simulink model "ARDroneWPTracking"  (R2014a)
settings: Solver=ode1  StartTime=0.0  StopTime=inf  FixedStep=sampleTime  RelTol=1e-3
values from neighbouring files (symbols this model uses):
  sampleTime = 0.04    [start.m]
  waypoints = getWaypoints()    [start.m]
undefined symbols (not defined in the file or in its folder): Standard_Devices, UDP_Protocol
libraries: ARBlocks x2, rtwinlib x1
CloseFcn:
  | rtwprivate ssgencode ModelCloseRequest Good_NL_model
settings Model: SimulationMode=external  ExtModeTrigDuration=100000  Creator=Paul  LastModifiedBy=Django
settings DataIOCC: SignalLoggingSaveFormat=ModelDataLogs  TimeSaveName=time
settings OptimizationCC: ExpressionDepthLimit=2147483647  InitFltsAndDblsToZero=on
settings DebuggingCC: UnderspecifiedInitializationDetection=Classic  FcnCallInpInsideContextMsg=UseLocalSettings  StateNameClashWarn=warning
settings HardwareCC: ProdIntDivRoundTo=Zero  ProdEndianess=LittleEndian  ProdHWDeviceType=Generic->32-bit x86 compatible
settings RTWCC: SystemTargetFile=rtwin.tlc  TemplateMakefile=rtwin.tmf  Description=Real-Time Windows Target  ProcessScript=rtwin_make_rtw_hook  RTWCompilerOptimization=On
settings CodeAppCC: MaxIdLength=95
settings RTWinTargetCC: TargetLibSuffix=_rtwin.lib  TargetPreCompLibLocation=E:\Installationposition\InstallPath\MATLAB\MATLAB2014a\toolbox\rtw\targets\rtwin\lib\win64

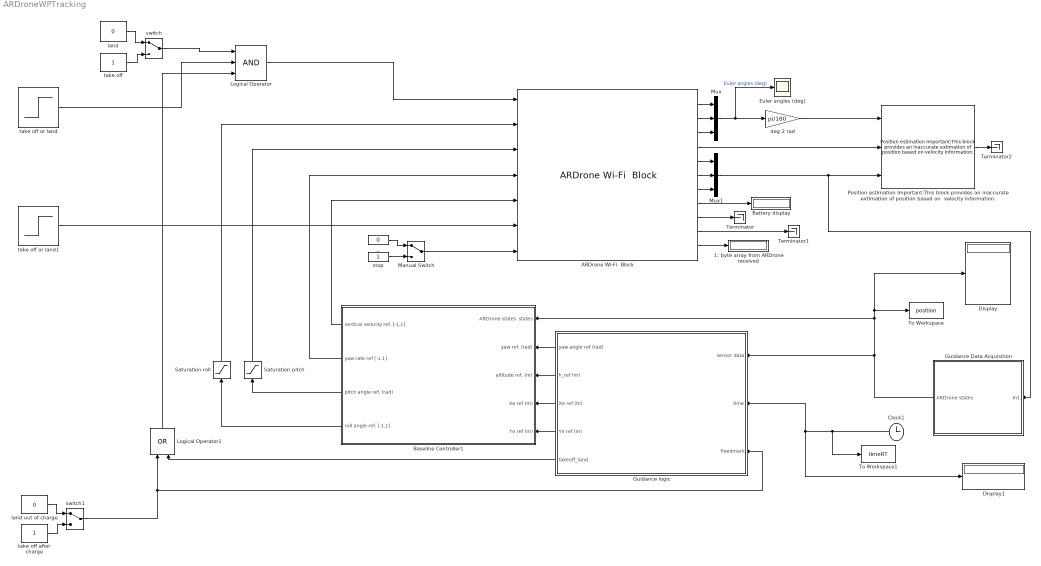
== system ARDroneWPTracking ==
  "1: byte array from ARDrone received " : Display
  ARDrone Wi-Fi  Block : ARBlocks/ARDrone Wi-Fi  Block
  Baseline Controller1 : Subsystem  AncestorBlock=ARBlocks/Baseline Controller
  Battery display : Display
  Clock1 : Clock
  Display : Display
  Display1 : Display
  Euler angles (deg) : Scope
      settings: YMin=-10  YMax=120  MaxDataPoints=500000
  Guidance Data Acquisition : Subsystem  AncestorBlock=ARBlocks/Guidance Data Acquisition
  Guidance logic : Subsystem  AncestorBlock=ARBlocks/Guidance logic
  Logical Operator : Logic  Inputs=3  AllPortsSameDT=off  OutDataTypeStr=boolean
  Logical Operator1 : Logic  Operator=OR  AllPortsSameDT=off  OutDataTypeStr=boolean
  Manual Switch : ManualSwitch
  Mux : Mux  Inputs=3
  Mux1 : Mux  Inputs=3
  "Position estimation Important:This block provides an inaccurate extimation of position based on  velocity information. " : ARBlocks/Position estimation Important:This block provides an  inaccurate extimation of position  based on  velocity information. 
  Saturation pitch : Saturate  UpperLimit=0.08  LowerLimit=-0.1
  Saturation roll : Saturate  UpperLimit=0.05  LowerLimit=-0.1
  Terminator : Terminator
  Terminator1 : Terminator
  Terminator2 : Terminator
  To Workspace : ToWorkspace  VariableName=position  SaveFormat=Structure With Time  SampleTime=sampleTime
  To Workspace1 : ToWorkspace  VariableName=timeRT  SampleTime=sampleTime
  _ : Constant  Value=0
  deg 2 rad : Gain  Gain=pi/180
  land : Constant  Value=0
  land out of charge : Constant  Value=0
  stop : Constant
  switch : ManualSwitch
  switch1 : ManualSwitch
  take off : Constant
  take off after charge : Constant
  take off or land : Step  Time=5  SampleTime=0
  take off or land1 : Step  Time=10  SampleTime=0
  wires:
  _/1 -> Manual Switch/1
  stop/1 -> Manual Switch/2
  Logical Operator/1 -> ARDrone Wi-Fi  Block/1
  take off or land1/1 -> ARDrone Wi-Fi  Block/6
  Manual Switch/1 -> ARDrone Wi-Fi  Block/7
  ARDrone Wi-Fi  Block/1 -> Mux/1
  ARDrone Wi-Fi  Block/2 -> Mux/2
  ARDrone Wi-Fi  Block/5 -> Mux1/1
  ARDrone Wi-Fi  Block/6 -> Mux1/2
  ARDrone Wi-Fi  Block/7 -> Mux1/3
  Mux/1 -> Euler angles (deg)/1, deg 2 rad/1  "Euler angles (deg)"
  ARDrone Wi-Fi  Block/8 -> Battery display/1
  Baseline Controller1/1(vertical velocity ref. [-1,1]) -> ARDrone Wi-Fi  Block/5
  Baseline Controller1/3(pitch angle ref. (rad)) -> Saturation pitch/1
  "Position estimation Important:This block provides an inaccurate extimation of position based on  velocity information. "/1 -> Terminator2/1
  deg 2 rad/1 -> "Position estimation Important:This block provides an inaccurate extimation of position based on  velocity information. "/1
  ARDrone Wi-Fi  Block/4 -> "Position estimation Important:This block provides an inaccurate extimation of position based on  velocity information. "/2
  Mux1/1 -> Guidance Data Acquisition/1(In1), "Position estimation Important:This block provides an inaccurate extimation of position based on  velocity information. "/3
  Clock1/1 -> To Workspace1/1, Display1/1, Guidance logic/2(time)
  Baseline Controller1/4(roll angle ref. [-1,1]) -> Saturation roll/1
  ARDrone Wi-Fi  Block/3 -> Mux/3
  Guidance logic/2(h_ref (m)) -> Baseline Controller1/3(altitude ref. (m))
  Guidance logic/4(Ye ref (m)) -> Baseline Controller1/5(Ye ref (m))
  Guidance logic/1(yaw angle ref (rad)) -> Baseline Controller1/2(yaw ref. (rad))
  ARDrone Wi-Fi  Block/9 -> Terminator/1
  ARDrone Wi-Fi  Block/10 -> Terminator1/1
  ARDrone Wi-Fi  Block/11 -> "1: byte array from ARDrone received "/1
  Baseline Controller1/2(yaw rate ref [-1,1]) -> ARDrone Wi-Fi  Block/4
  Guidance Data Acquisition/1(ARDrone states) -> Guidance logic/1(sensor data), Baseline Controller1/1("ARDrone states  states "), Display/1, To Workspace/1
  land/1 -> switch/1
  take off/1 -> switch/2
  switch/1 -> Logical Operator/1
  take off or land/1 -> Logical Operator/2
  Guidance logic/3(Xe ref (m)) -> Baseline Controller1/4(Xe ref (m))
  Logical Operator1/1 -> Logical Operator/3
  Saturation pitch/1 -> ARDrone Wi-Fi  Block/3
  Saturation roll/1 -> ARDrone Wi-Fi  Block/2
  land out of charge/1 -> switch1/1
  take off after charge/1 -> switch1/2
  switch1/1 -> Logical Operator1/1, Guidance logic/3(fixedmark)
  Guidance logic/5(takeoff_land) -> Logical Operator1/2

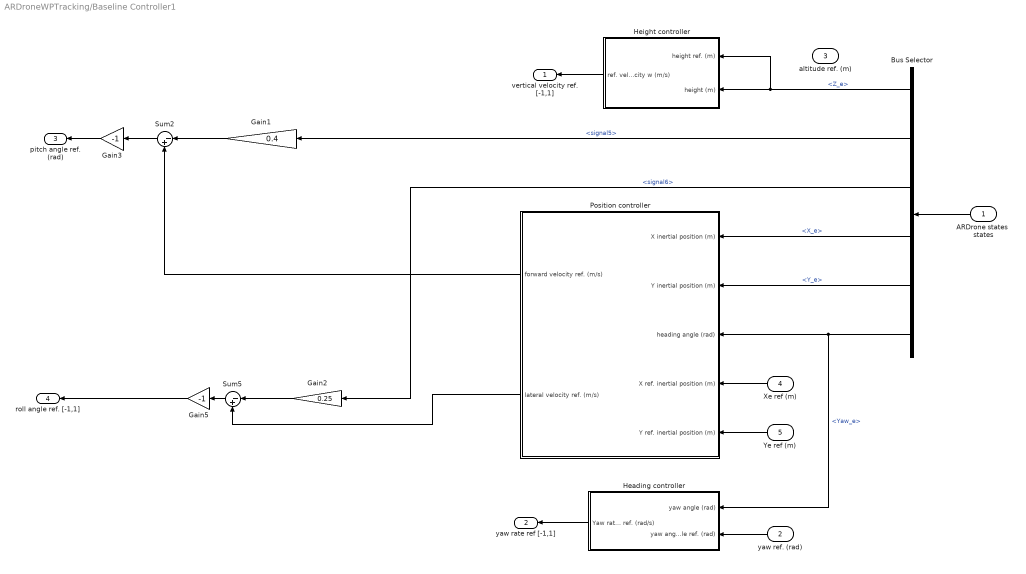
== system ARDroneWPTracking/Baseline Controller1 ==
  "ARDrone states  states " : Inport
  yaw ref. (rad) : Inport  Port=2
  altitude ref. (m) : Inport  Port=3
  Xe ref (m) : Inport  Port=4
  Ye ref (m) : Inport  Port=5
  Bus Selector : BusSelector  OutputSignals=Z_e,signal5,signal6,X_e,Y_e,Yaw_e
  Gain1 : Gain  Gain=0.4
  Gain2 : Gain  Gain=0.25
  Gain3 : Gain  Gain=-1
  Gain5 : Gain  Gain=-1
  Heading controller : Subsystem
  "Height controller " : Subsystem
  Position controller : Subsystem
  Sum2 : Sum  Inputs=|-+
  Sum5 : Sum  Inputs=|-+
  vertical velocity ref. [-1,1] : Outport
  yaw rate ref [-1,1] : Outport  Port=2
  pitch angle ref. (rad) : Outport  Port=3
  roll angle ref. [-1,1] : Outport  Port=4
  wires:
  Ye ref (m)/1 -> Position controller/5(Y ref. inertial position (m))
  Xe ref (m)/1 -> Position controller/4(X ref. inertial position (m))
  Bus Selector/5 -> Position controller/2(Y inertial position (m))  "<Y_e>"
  Bus Selector/4 -> Position controller/1(X inertial position (m))  "<X_e>"
  Heading controller/1(Yaw rate ref. (rad/s)) -> yaw rate ref [-1,1]/1
  yaw ref. (rad)/1 -> Heading controller/2(yaw angle ref. (rad))
  Bus Selector/2 -> Gain1/1  "<signal5>"
  Gain5/1 -> roll angle ref. [-1,1]/1
  "Height controller "/1(ref. velocity w (m/s)) -> vertical velocity ref. [-1,1]/1
  Bus Selector/1 -> "Height controller "/1(height ref. (m)), "Height controller "/2(height (m))  "<Z_e>"
  "ARDrone states  states "/1 -> Bus Selector/1
  Bus Selector/6 -> Position controller/3(heading angle (rad)), Heading controller/1(yaw angle (rad))  "<Yaw_e>"
  Sum2/1 -> Gain3/1
  Gain1/1 -> Sum2/1
  Gain3/1 -> pitch angle ref. (rad)/1
  Position controller/1(forward velocity ref. (m/s)) -> Sum2/2
  Sum5/1 -> Gain5/1
  Bus Selector/3 -> Gain2/1  "<signal6>"
  Gain2/1 -> Sum5/1
  Position controller/2(lateral velocity ref. (m/s)) -> Sum5/2

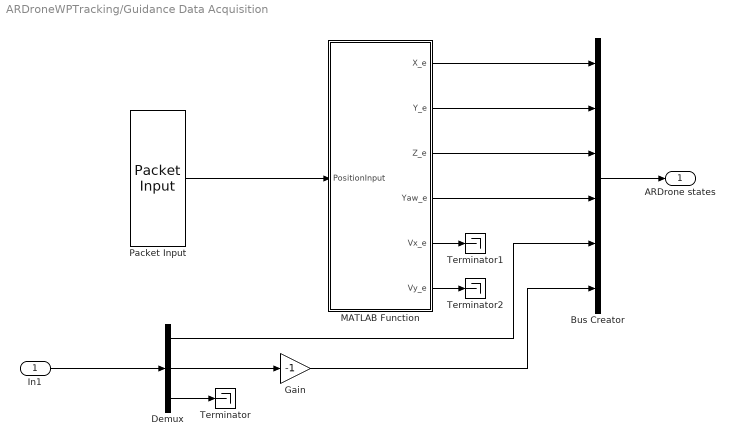
== system ARDroneWPTracking/Guidance Data Acquisition ==
  In1 : Inport
  Bus Creator : BusCreator  Inputs=6
  Demux : Demux  Outputs=3
  Gain : Gain  Gain=-1
  MATLAB Function : MATLAB Function  TreatAsAtomicUnit=on
  Packet Input : rtwinlib/Packet Input  SampleTime=sampleTime  MaxMissedTicks=1  ShowMissedTicks=off  YieldWhenWaiting=on  DrvName=Standard_Devices/UDP_Protocol  DrvAddress=5500  DrvOptions=[3215458314 5500]  PacketSize=32  DataTypes='4*double'  ShowReady=off  ShowError=off  PacketID=1  ByteOrder=2  ShowTimestamp=off
      settings: AttributesFormatString=Standard Devices\nUDP Protocol [157Ch]
  Terminator : Terminator
  Terminator1 : Terminator
  Terminator2 : Terminator
  ARDrone states : Outport
  wires:
  Demux/3 -> Terminator/1
  Demux/2 -> Gain/1
  In1/1 -> Demux/1
  Gain/1 -> Bus Creator/6
  Demux/1 -> Bus Creator/5
  Bus Creator/1 -> ARDrone states/1
  MATLAB Function/4(Yaw_e) -> Bus Creator/4
  Packet Input/1 -> MATLAB Function/1(PositionInput)
  MATLAB Function/1(X_e) -> Bus Creator/1
  MATLAB Function/2(Y_e) -> Bus Creator/2
  MATLAB Function/3(Z_e) -> Bus Creator/3
  MATLAB Function/5(Vx_e) -> Terminator1/1
  MATLAB Function/6(Vy_e) -> Terminator2/1

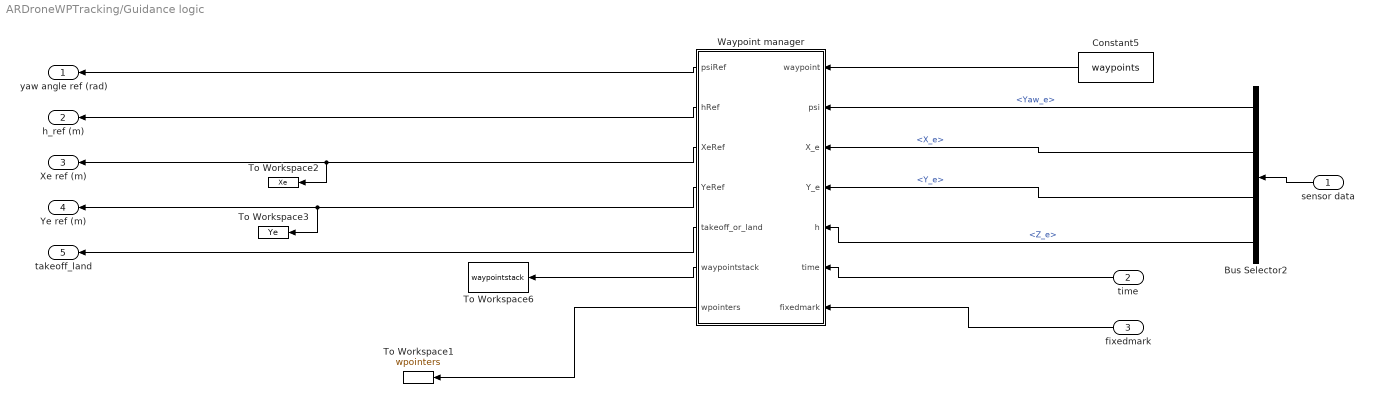
== system ARDroneWPTracking/Guidance logic ==
  sensor data : Inport
  time : Inport  Port=2
  fixedmark : Inport  Port=3
  Bus Selector2 : BusSelector  OutputSignals=Yaw_e,X_e,Y_e,Z_e
  Constant5 : Constant  Value=waypoints  VectorParams1D=off
  To Workspace1 : ToWorkspace  VariableName=wpointers  SampleTime=sampleTime
  To Workspace2 : ToWorkspace  VariableName=Xe  SampleTime=sampleTime
  To Workspace3 : ToWorkspace  VariableName=Ye  SampleTime=sampleTime
  To Workspace6 : ToWorkspace  VariableName=waypointstack  SampleTime=sampleTime
  "Waypoint manager " : MATLAB Function  TreatAsAtomicUnit=on
  yaw angle ref (rad) : Outport
  h_ref (m) : Outport  Port=2
  Xe ref (m) : Outport  Port=3
  Ye ref (m) : Outport  Port=4
  takeoff_land : Outport  Port=5
  wires:
  Constant5/1 -> "Waypoint manager "/1(waypoint)
  "Waypoint manager "/1(psiRef) -> yaw angle ref (rad)/1
  time/1 -> "Waypoint manager "/6(time)
  Bus Selector2/4 -> "Waypoint manager "/5(h)  "<Z_e>"
  "Waypoint manager "/4(YeRef) -> To Workspace3/1, Ye ref (m)/1
  "Waypoint manager "/3(XeRef) -> To Workspace2/1, Xe ref (m)/1
  "Waypoint manager "/2(hRef) -> h_ref (m)/1
  Bus Selector2/1 -> "Waypoint manager "/2(psi)  "<Yaw_e>"
  sensor data/1 -> Bus Selector2/1
  Bus Selector2/3 -> "Waypoint manager "/4(Y_e)  "<Y_e>"
  Bus Selector2/2 -> "Waypoint manager "/3(X_e)  "<X_e>"
  "Waypoint manager "/5(takeoff_or_land) -> takeoff_land/1
  "Waypoint manager "/6(waypointstack) -> To Workspace6/1
  fixedmark/1 -> "Waypoint manager "/7(fixedmark)
  "Waypoint manager "/7(wpointers) -> To Workspace1/1

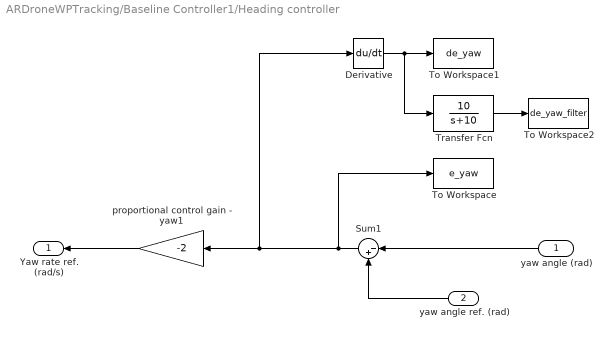
== system ARDroneWPTracking/Baseline Controller1/Heading controller ==
  yaw angle (rad) : Inport
  yaw angle ref. (rad) : Inport  Port=2
  Derivative : Derivative
  Sum1 : Sum  Inputs=|-+
  To Workspace : ToWorkspace  VariableName=e_yaw  SampleTime=-1
  To Workspace1 : ToWorkspace  VariableName=de_yaw  SampleTime=-1
  To Workspace2 : ToWorkspace  VariableName=de_yaw_filter  SampleTime=-1
  Transfer Fcn : TransferFcn  Numerator=[10]  Denominator=[1 10]
  proportional control gain - yaw1 : Gain  Gain=-2
  Yaw rate ref. (rad/s) : Outport
  wires:
  yaw angle ref. (rad)/1 -> Sum1/2
  yaw angle (rad)/1 -> Sum1/1
  proportional control gain - yaw1/1 -> Yaw rate ref. (rad/s)/1
  Sum1/1 -> proportional control gain - yaw1/1, Derivative/1, To Workspace/1
  Derivative/1 -> Transfer Fcn/1, To Workspace1/1
  Transfer Fcn/1 -> To Workspace2/1

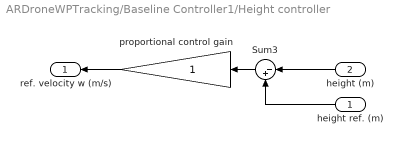
== system ARDroneWPTracking/Baseline Controller1/Height controller  ==
  height ref. (m) : Inport
  height (m) : Inport  Port=2
  Sum3 : Sum  Inputs=|-+
  proportional control gain : Gain
  ref. velocity w (m/s) : Outport
  wires:
  height ref. (m)/1 -> Sum3/2
  height (m)/1 -> Sum3/1
  Sum3/1 -> proportional control gain/1
  proportional control gain/1 -> ref. velocity w (m/s)/1

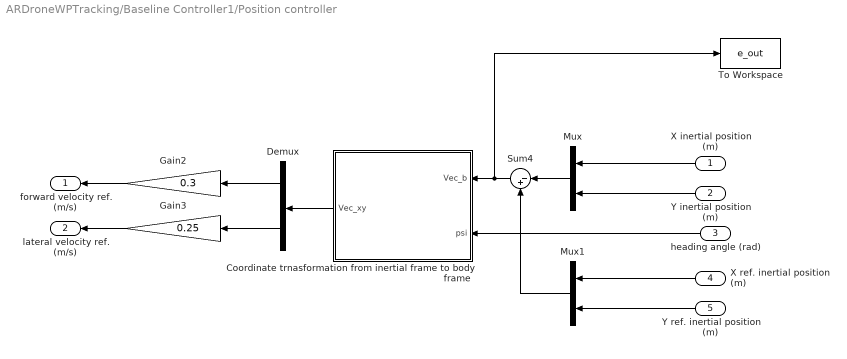
== system ARDroneWPTracking/Baseline Controller1/Position controller ==
  X inertial position (m) : Inport
  Y inertial position (m) : Inport  Port=2
  heading angle (rad) : Inport  Port=3
  X ref. inertial position (m) : Inport  Port=4
  Y ref. inertial position (m) : Inport  Port=5
  "Coordinate trnasformation from inertial frame to body frame " : MATLAB Function  TreatAsAtomicUnit=on
  Demux : Demux  Outputs=2
  Gain2 : Gain  Gain=0.3
  Gain3 : Gain  Gain=0.25
  Mux : Mux  Inputs=2
  Mux1 : Mux  Inputs=2
  Sum4 : Sum  Inputs=|-+
  To Workspace : ToWorkspace  VariableName=e_out  SampleTime=-1
  forward velocity ref. (m/s) : Outport
  lateral velocity ref. (m/s) : Outport  Port=2
  wires:
  Gain3/1 -> lateral velocity ref. (m/s)/1
  Demux/2 -> Gain3/1
  Demux/1 -> Gain2/1
  Y ref. inertial position (m)/1 -> Mux1/2
  X ref. inertial position (m)/1 -> Mux1/1
  Mux/1 -> Sum4/1
  X inertial position (m)/1 -> Mux/1
  Y inertial position (m)/1 -> Mux/2
  Sum4/1 -> To Workspace/1, "Coordinate trnasformation from inertial frame to body frame "/1(Vec_b)
  Mux1/1 -> Sum4/2
  "Coordinate trnasformation from inertial frame to body frame "/1(Vec_xy) -> Demux/1
  heading angle (rad)/1 -> "Coordinate trnasformation from inertial frame to body frame "/2(psi)
  Gain2/1 -> forward velocity ref. (m/s)/1

== matlab function ARDroneWPTracking/Baseline Controller1/Position controller/Coordinate trnasformation from inertial frame to body frame  ==
  data: Vec_b input; Vec_xy output; psi input
function Vec_xy  = fcn(Vec_b , psi)
%#codegen
T = [cos(psi) sin(psi) ; -sin(psi) cos(psi)] ; 
Vec_xy = T*Vec_b(1:2,1);

== matlab function ARDroneWPTracking/Guidance Data Acquisition/MATLAB Function ==
  data: X_e output; PositionInput input; Y_e output; Z_e output; Yaw_e output; Vx_e output; Vy_e output
function [X_e,Y_e,Z_e,Yaw_e,Vx_e,Vy_e] = fcn(PositionInput)
%#codegen
persistent xPre;
if isempty(xPre)
    xPre = 0;
end

persistent yPre;
if isempty(yPre)
    yPre = 0;
end

X_e = PositionInput(1)/1000;
Y_e = PositionInput(2)/1000;
Z_e = PositionInput(3)/1000;
Yaw_e = PositionInput(4);

Vx_e = (X_e - xPre)/0.065;
Vy_e = (Y_e - yPre)/0.065;
xPre = X_e;
yPre = Y_e;
end

== matlab function ARDroneWPTracking/Guidance logic/Waypoint manager  ==
  data: psiRef output; hRef output; waypoint input; psi input; X_e input; Y_e input; h input; XeRef output; YeRef output; time input; takeoff_or_land output; waypointstack output; fixedmark input; wpointers output
function [psiRef,hRef,XeRef,YeRef,takeoff_or_land,waypointstack,wpointers]       = fcn(waypoint, psi, X_e,Y_e, h, time,fixedmark )
%#codegen
% 航点矩阵每一列包括航点位置，航向角,飞机在该航点的等待时间.
%%%%%%%%%%%%%%%%%%%%%%%%%%%%%%%%%%%%%%%%%%%%%%%%%%%%%%%%%%%%%%%%%%%%%%%%%%%
% 定义全局矩阵保存航点信息，相当于一个栈
persistent Gwaypoint;
if isempty(Gwaypoint)
    Gwaypoint = [waypoint zeros(5,10)];
end

% 航点数
nPoints = size(Gwaypoint, 2) - 10;

% 故障标志
persistent charge;
if isempty(charge)
    charge = 0;
end

% 航点栈指针，总指向下一个目标位置
persistent wpointer;
if isempty(wpointer)
    wpointer = nPoints;
end

% 计时器，记录飞机到达航点的时刻
persistent t0 ;
if isempty(t0)
    t0 = 0;
end

% 记录故障发生时的地点
persistent OutofCharge ;
if isempty(OutofCharge)
    OutofCharge = [0,0,0,0,2]';
end

% 记录故障处理中心地点及处理时间
persistent chargeStation ;
if isempty(chargeStation)
    chargeStation = [-0.5,0.5,1,0,8]';
end

% 飞机起飞\降落标志
persistent takeoff_land ;
if isempty(takeoff_land)
    takeoff_land = 1;
end

if (fixedmark == 1)
    takeoff_land = 1;
end
%%%%%%%%%%%%%%%%%%%%%%%%%%%%%%%%%%%%%%%%%%%%%%%%%%%%%%%%%%%%%%%%%%%%%%%%%%%
%%%%%%%%%%%%%%%%%%%%%%%%%%%%%%%%%%%%%%%%%%%%%%%%%%%%%%%%%%%%%%%%%%%%%%%%%%%
% 只有故障标志为0时才判断是否有故障发生

if(charge == 0)
    % 假设飞机在某个时间区间出现故障
if(time > 24 && time < 24.3)
    charge = 1; % 故障标志置为1
    % 立即记录故障发生地点
    OutofCharge(1) = X_e;
    OutofCharge(2) = Y_e;
    OutofCharge(3) = h;
    % 使故障发生地点入航点栈，修理完成后在修理中心处悬停一会儿，待稳定后飞向故障地点
    wpointer = wpointer + 1;
    Gwaypoint(:,wpointer) = OutofCharge;
%   Gwaypoint = [Gwaypoint(:,1:wpointer-1) OutofCharge];
    % 使故障处理中心地点入航点栈，修理完成后先在这个点悬停一会儿
    wpointer = wpointer + 1;
    Gwaypoint(:,wpointer) = chargeStation;
    % 使故障处理中心地点入航点栈，检测到故障后立即飞向这个点
    wpointer = wpointer + 1;
    Gwaypoint(:,wpointer) = chargeStation;
    %Gwaypoint = [Gwaypoint(:,1:wpointer-1) chargeStation];
%     Gwaypoint
%     % 再次使故障发生地点入航点栈，先让飞机在故障点停一会儿
%     wpointer = wpointer + 1;
%     Gwaypoint(:,wpointer) = OutofCharge;
end
end

%%%%%%%%%%%%%%%%%%%%%%%%%%%%%%%%%%%%%%%%%%%%%%%%%%%%%%%%%%%%%%%%%%%%%%%%%%%%%%%%%%%%%%%%%%%%%%%%%%

if ( norm([X_e,Y_e]' - Gwaypoint(1:2, wpointer) )< 0.3 && ...
        norm(h - Gwaypoint(3, wpointer)) < 0.3  && norm(psi - Gwaypoint(4, wpointer) )< 5*pi/180 )
   if(charge == 1)
    % 如果故障标志为1，则当前到达的航点就是故障处理中心
%     if(wpointer > 0)
%         
%         if (t0 ==0)
%             % 立即记录到达时间
%             t0 = time;
%         else
%             if (time - t0 > Gwaypoint(5, wpointer)) 
%                 % 故障处理结束，使航点指针指向下一个航点，计时器清零，故障状态清零
%                 wpointer = wpointer - 1;
%                 t0 = 0;
%                 charge = 0;
%             end
%         end
%     end
      wpointer = wpointer - 1;
      charge = 0;
      takeoff_land = 0;
   end
   if(charge == 0)
    % 如果故障状态为0，则当前到达的航点为任务航点
    if(wpointer > 1)
       % 当前航点不是最后一个航点，不需要将基站（home）位置入栈
        if (t0 ==0)
             % 立即记录到达时间
            t0 = time;
        else
           if (time - t0 > Gwaypoint(5, wpointer))  
              % 在该航点的任务结束，使航点指针指向下一个航点，计时器清零
              wpointer = wpointer - 1;
              t0 = 0;
           end
                
         end
    end 
    if(wpointer == 1)
        % 当前航点为最后一个航点，执行完该航点任务飞机要返航回基站
         if (t0 ==0)
             % 立即记录到达时间
            t0 = time;
        else
            if (time - t0 > Gwaypoint(5, wpointer))          
                    t0 = 0;
                    takeoff_land = 0;                   
            end               
         end 
    end
    end     
end
%% Outputs:
    hRef = Gwaypoint(3, wpointer) ;
    psiRef = Gwaypoint(4, wpointer) ;
    XeRef = Gwaypoint(1, wpointer) ;
    YeRef = Gwaypoint(2, wpointer) ;
    takeoff_or_land = takeoff_land;
    waypointstack = Gwaypoint;
    wpointers = wpointer;










% %#codegen
% 
% % Waypoint matrix contains final position, orientatoin, and waiting time.
% 
% % Number of waypoints
% nPoints = size(waypoint, 2) ;
% 
% % Persitent variable used to keep trak of next waypoint
% persistent wpointer;
% 
% % Time zero for each waypoint. This is used to wait at a desired position.
% persistent t0 ;
% 
% % Init. persistent variables
% if isempty(wpointer)
%     wpointer = 1;
% end
% 
% if isempty(t0)
%     t0 = 0;
% end
% 
% % A waypoint is reached if the distance between the desired waypoint and 
% % the vehicle is less than 0.3 m in the XY plane, less than 0.3 m in height, 
% % and less than 5 degrees in  heading. 
% 
% if ( norm([X_e,Y_e]' - waypoint(1:2, wpointer) )< 0.3 && ...
%         norm(h - waypoint(3, wpointer)) < 0.3  && norm(psi - waypoint(4, wpointer) )< 5*pi/180   )
%     
%     if(wpointer ~= nPoints)
%         
%         if (t0 ==0)
%             t0 = time;
%         else
%             if (time - t0 > waypoint(5, wpointer))
%                 
%                  if(wpointer < nPoints)
%                     wpointer = wpointer+ 1;
%                     t0 = 0;
%                  end
%                 
%             end
%         end
%         
%              
%     end
%     
%        
%     
% end
% 
% 
% %% Outputs:
% hRef = waypoint(3, wpointer) ;
% psiRef = waypoint(4, wpointer) ;
% XeRef = waypoint(1, wpointer) ;
% YeRef = waypoint(2, wpointer) ;
% waypointNumber = wpointer ;
